simulink model "ThreePhase_Fullwave"  (R2020a)
settings: Solver=VariableStepAuto  StartTime=0.0  StopTime=0.01  RelTol=1e-3
libraries: powerlib x16
settings Model: Creator=Naeem Mohammad  LastModifiedBy=Naeem Mohammad

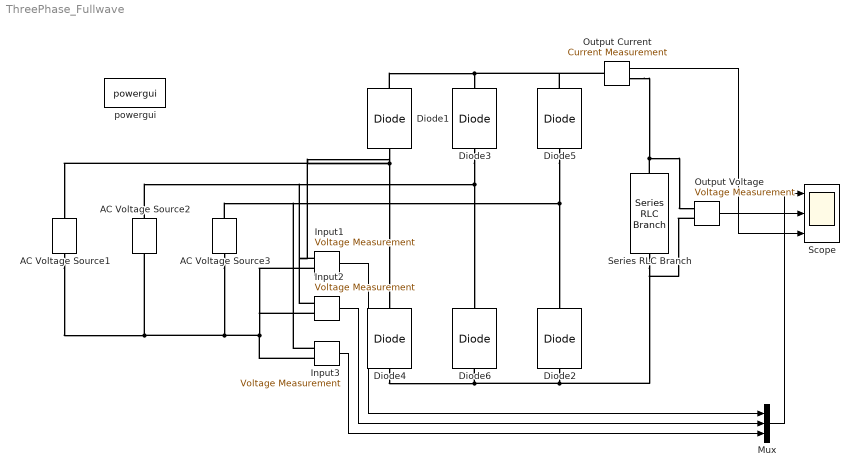
== system ThreePhase_Fullwave ==
  AC Voltage Source3 : powerlib/Electrical Sources/AC Voltage Source  Amplitude=110  Phase=240  Frequency=60  SampleTime=0  Measurements=None  BusType=swing  Pref=10e3  Qref=0  Qmin=-inf  Qmax=+inf
  AC Voltage Source1 : powerlib/Electrical Sources/AC Voltage Source  Amplitude=110  Phase=0  Frequency=60  SampleTime=0  Measurements=None  BusType=swing  Pref=10e3  Qref=0  Qmin=-inf  Qmax=+inf
  AC Voltage Source2 : powerlib/Electrical Sources/AC Voltage Source  Amplitude=110  Phase=120  Frequency=60  SampleTime=0  Measurements=None  BusType=swing  Pref=10e3  Qref=0  Qmin=-inf  Qmax=+inf
  Diode{1..6} (6 alike) : powerlib/Power Electronics/Diode  Ron=0.001  Lon=0  Vf=0.8  IC=0  UseSnubber=0  Rs=500  Cs=250e-9  Measurements=off
  Input1 : powerlib/Measurements/Voltage Measurement  PhasorSimulation=off  OutputType=Complex  PSBequivalent=0
  Input2 : powerlib/Measurements/Voltage Measurement  PhasorSimulation=off  OutputType=Complex  PSBequivalent=0
  Input3 : powerlib/Measurements/Voltage Measurement  PhasorSimulation=off  OutputType=Complex  PSBequivalent=0
  Mux : Mux  Inputs=3
  Output Voltage : powerlib/Measurements/Voltage Measurement  PhasorSimulation=off  OutputType=Complex  PSBequivalent=0
  Output Current : powerlib/Measurements/Current Measurement  PhasorSimulation=off  OutputType=Complex  PSBequivalent=0
  Scope : Scope  NumInputPorts=3
  Series RLC Branch : powerlib/Elements/Series RLC Branch  LConnTagsString=__new0  RConnTagsString=__new0  BranchType=R  Resistance=100  Inductance=1e-3  SetiL0=off  InitialCurrent=0  Capacitance=1e-6  Setx0=off  InitialVoltage=0  Measurements=None
  powergui : powerlib/powergui  Priority=1  SimulationMode=Discrete  SampleTime=50e-6  frequency=60  Iterations=50  frequencyindice=0  Pbase=100e6  ErrMax=1e-4  UnitsV=kV  UnitsW=MW  buscounter=0  FunctionMessages=off  echomessages=off  EnableUseOfTLC=off  CurrentSourceSwitches=off  DisableSnubberDevices=off  DisableRonSwitches=off  DisableVfSwitches=off  DisplayEquations=off  AutomaticDiscreteSolvers=off  SolverType=Tustin/Backward Euler (TBE)  Interpol=off  ExternalGateDelay=off  methode=off  Ts=100  x0status=blocks  SPID=on  SwTol=0  HookPort=off  NonlinearTolerance=1e-4  nMaxIteration=100  ContinueOnMaxIteration=off  RestoreLinks=warning  ResistiveCurrentMeasurement=off  Frange=[0:2:500]  Ylog=off  Xlog=on  ShowGrid=off  save=off  variable=ZData  structure=0  ZoomFFT=off  StartTime=0.0  cycles=1  DisplayStyle=1  fundamental=60  FreqAxis=off  MaxFrequency=1000  frequencyindicesteady=1  RmsSteady=1  display=off
  wires:
  Output Voltage/1 -> Scope/2
  Input1/1 -> Mux/1
  Input2/1 -> Mux/2
  Input3/1 -> Mux/3
  Mux/1 -> Scope/1
  Output Current/1 -> Scope/3
  connections:
  Diode1/RConn1 -- Output Current/LConn1 -- Diode5/RConn1 -- Diode3/RConn1
  Diode1/LConn1 -- Input1/LConn1 -- AC Voltage Source1/RConn1 -- Diode4/RConn1
  Diode3/LConn1 -- Input2/LConn1 -- AC Voltage Source2/RConn1 -- Diode6/RConn1
  Diode5/LConn1 -- AC Voltage Source3/RConn1 -- Input3/LConn1 -- Diode2/RConn1
  Diode4/LConn1 -- Output Voltage/LConn2 -- Series RLC Branch/RConn1 -- Diode2/LConn1 -- Diode6/LConn1
  AC Voltage Source1/LConn1 -- AC Voltage Source3/LConn1 -- Input2/LConn2 -- Input1/LConn2 -- Input3/LConn2 -- AC Voltage Source2/LConn1
  Series RLC Branch/LConn1 -- Output Voltage/LConn1 -- Output Current/RConn1
